simulink model "prac1s2022a"  (R2022a)
settings: Solver=FixedStepAuto  StartTime=0.0  StopTime=50  FixedStep=1e-4  RelTol=1e-3
undefined symbols (not defined in the file): A, B, C, D, K1, K2, K3, x0
settings Model: Creator=86156  LastModifiedBy=86156
settings ModelReferenceCC: EnableRefExpFcnMdlSchedulingChecks=off
settings RTWCC: Description=Generic Real-Time Target  GPUComputeCapability=5.0

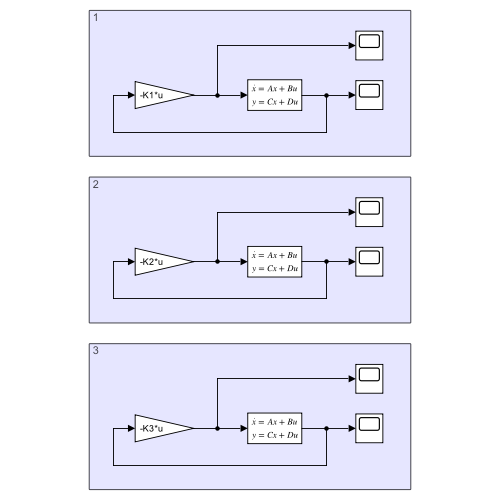
[thumbnail: Simulink's stored preview of the top-level diagram]
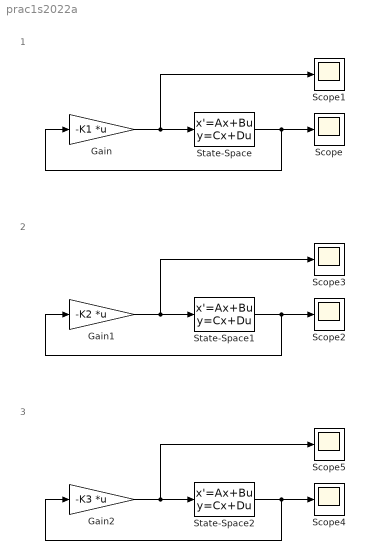
== system prac1s2022a ==
  note: 1
  note: 2
  note: 3
  Gain : Gain  Gain=-K1  Multiplication=Matrix(K*u)
  Gain1 : Gain  Gain=-K2  Multiplication=Matrix(K*u)
  Gain2 : Gain  Gain=-K3  Multiplication=Matrix(K*u)
  Scope{,1..5} (6 alike) : Scope
  State-Space : StateSpace  A=A  B=B  C=C  D=D  InitialCondition=x0
  State-Space1 : StateSpace  A=A  B=B  C=C  D=D  InitialCondition=x0
  State-Space2 : StateSpace  A=A  B=B  C=C  D=D  InitialCondition=x0
  wires:
  State-Space/1 -> Gain/1, Scope/1
  Gain/1 -> Scope1/1, State-Space/1
  State-Space1/1 -> Gain1/1, Scope2/1
  Gain1/1 -> Scope3/1, State-Space1/1
  State-Space2/1 -> Gain2/1, Scope4/1
  Gain2/1 -> Scope5/1, State-Space2/1
